simulink model "Lab1_works_ish"  (R2018a)
settings: Solver=VariableStepAuto  StartTime=0.0  StopTime=100  RelTol=1e-3
values from neighbouring files (symbols this model uses):
  Ac = [-(a*g*sqrt(2))/(2*sqrt((h10+h0)*g)*A) 0 ... (first row only)    [Lab1.m]    (also in LabB_FInal_version2.mat = [-0.0357235328446  0; 0.0357235328446  -0.0357235328446]; Untitled.m)
  Bc = [1/A ... (first row only)    [Lab1.m]    (also in LabB_FInal_version2.mat = [0.030303030303 0]; Untitled.m)
  C1 = [1 0]    [Lab1.m]    (also in LabB_FInal_version2.mat; Untitled.m)
  C2 = [0 1]    [Lab1.m]    (also in LabB_FInal_version2.mat; Untitled.m)
  K = K'    [Lab1.m]    (also in LabB_FInal_version2.mat = [5.99248777663 0.992989193414]; Untitled.m)
  v = 1:1:10    [Lab1.m]    (also in LabB_FInal_version2.mat = [1 2 3 4 5 6 7 8 9 10]; Untitled.m)
  vt = [21.18, 26.66 30.97, 34.28, 37.92, 39.73, 42.53, 45.45, 46.49, 47.67]    [Lab1.m]    (also in LabB_FInal_version2.mat = [21.18 26.66 30.97 34.28 37.92 39.73 42.53 45.45 46.49 47.67; Untitled.m)
settings Model: Creator=Scott  LastModifiedBy=oscbck-5

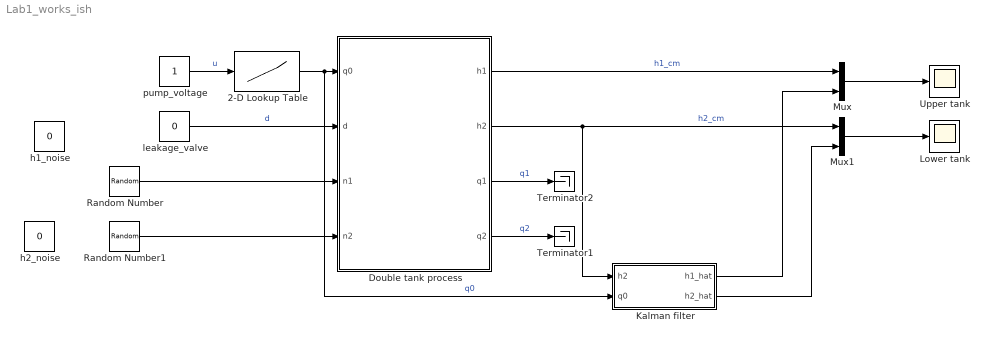
== system Lab1_works_ish ==
  2-D Lookup Table : Lookup_n-D  NumberOfTableDimensions=1  BreakpointsForDimension1=x  BreakpointsForDimension2=[1:3]  Table=y  RndMeth=Simplest  InputSameDT=on  mask{x=v, y=vt}
      mask prompts: x "Values on x-axis"; y "Values on y-axis"
  Double tank process : Subsystem  mask{At=33, Ao=0.17, hmax=15.5}
      mask prompts: At "Tank area (cm^2)"; Ao "Opening area (cm^2)"; hmax "Tank height (cm)"
      mask help: Double tank process parameters
  Kalman filter : Subsystem
  Lower tank : Scope
  Mux : Mux  Inputs=2
  Mux1 : Mux  Inputs=2
  Random Number : RandomNumber  Variance=0.1  SampleTime=0.1
  Random Number1 : RandomNumber  Variance=0.1  SampleTime=0.1
  Terminator1 : Terminator
  Terminator2 : Terminator
  Upper tank : Scope
  h1_noise : Constant  Value=0
  h2_noise : Constant  Value=0
  leakage_valve : Constant  Value=0
  pump_voltage : Constant
  wires:
  2-D Lookup Table/1 -> Kalman filter/2(q0), Double tank process/1(q0)  "q0"
  Double tank process/2(h2) -> Mux1/1, Kalman filter/1(h2)  "h2_cm"
  leakage_valve/1 -> Double tank process/2(d)  "d"
  pump_voltage/1 -> 2-D Lookup Table/1  "u"
  Double tank process/1(h1) -> Mux/1  "h1_cm"
  Double tank process/3(q1) -> Terminator2/1  "q1"
  Double tank process/4(q2) -> Terminator1/1  "q2"
  Mux/1 -> Upper tank/1
  Kalman filter/1(h1_hat) -> Mux/2
  Mux1/1 -> Lower tank/1
  Kalman filter/2(h2_hat) -> Mux1/2
  Random Number1/1 -> Double tank process/4(n2)
  Random Number/1 -> Double tank process/3(n1)

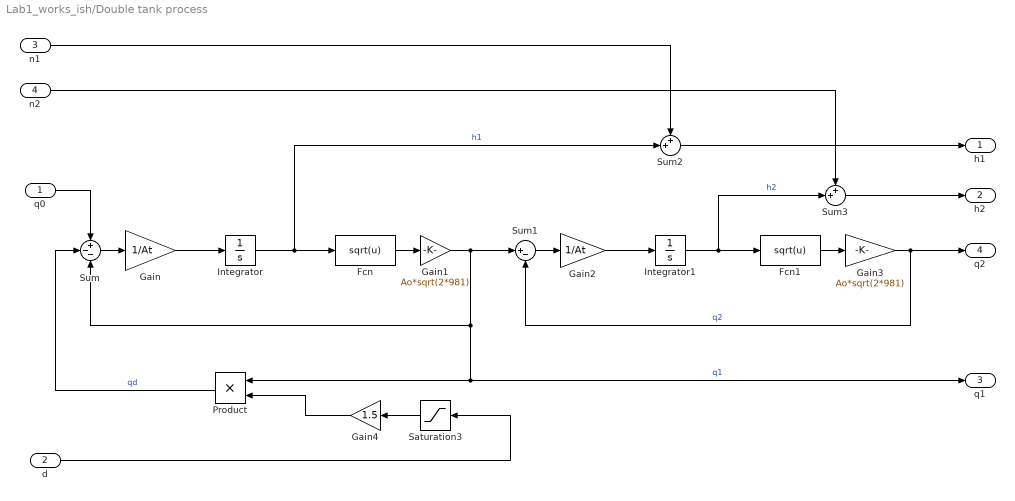
== system Lab1_works_ish/Double tank process ==
  q0 : Inport
  d : Inport  Port=2
  n1 : Inport  Port=3
  n2 : Inport  Port=4
  Fcn : Fcn  Expr=sqrt(u)
  Fcn1 : Fcn  Expr=sqrt(u)
  Gain : Gain  Gain=1/At
  Gain1 : Gain  Gain=Ao*sqrt(2*981)
  Gain2 : Gain  Gain=1/At
  Gain3 : Gain  Gain=Ao*sqrt(2*981)
  Gain4 : Gain  Gain=1.5
  Integrator : Integrator  LimitOutput=on  UpperSaturationLimit=hmax  LowerSaturationLimit=0
  Integrator1 : Integrator  LimitOutput=on  UpperSaturationLimit=hmax  LowerSaturationLimit=0
  Product : Product  RndMeth=Zero
  Saturation3 : Saturate  UpperLimit=1  LowerLimit=0
  Sum : Sum  Inputs=+--
  Sum1 : Sum  Inputs=|+-
  Sum2 : Sum  Inputs=++|
  Sum3 : Sum  Inputs=++|
  h1 : Outport
  h2 : Outport  Port=2
  q1 : Outport  Port=3
  q2 : Outport  Port=4
  wires:
  Sum/1 -> Gain/1
  Gain/1 -> Integrator/1
  Fcn/1 -> Gain1/1
  Gain1/1 -> Sum1/1, Product/1, q1/1, Sum/3  "q1"
  Sum1/1 -> Gain2/1
  Gain2/1 -> Integrator1/1
  Fcn1/1 -> Gain3/1
  Gain3/1 -> Sum1/2, q2/1  "q2"
  q0/1 -> Sum/1
  Integrator/1 -> Sum2/2, Fcn/1  "h1"
  Product/1 -> Sum/2  "qd"
  d/1 -> Saturation3/1
  Integrator1/1 -> Sum3/2, Fcn1/1  "h2"
  Saturation3/1 -> Gain4/1
  Gain4/1 -> Product/2
  Sum2/1 -> h1/1
  n1/1 -> Sum2/1
  Sum3/1 -> h2/1
  n2/1 -> Sum3/1

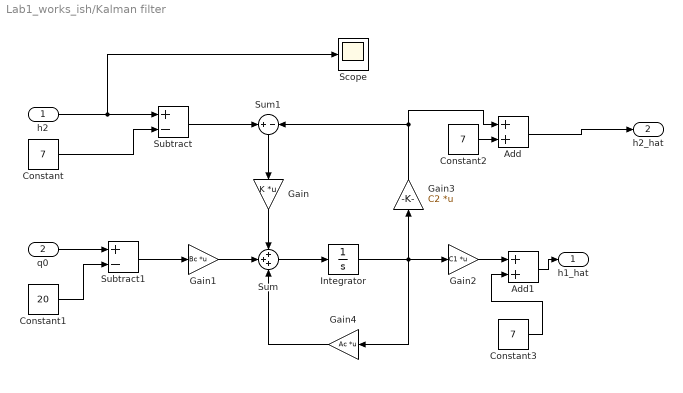
== system Lab1_works_ish/Kalman filter ==
  h2 : Inport
  q0 : Inport  Port=2
  Add : Sum
  Add1 : Sum
  Constant : Constant  Value=7
  Constant1 : Constant  Value=20
  Constant2 : Constant  Value=7
  Constant3 : Constant  Value=7
  Gain : Gain  Gain=K  Multiplication=Matrix(K*u)
  Gain1 : Gain  Gain=Bc  Multiplication=Matrix(K*u)
  Gain2 : Gain  Gain=C1  Multiplication=Matrix(K*u)
  Gain3 : Gain  Gain=C2  Multiplication=Matrix(K*u)
  Gain4 : Gain  Gain=Ac  Multiplication=Matrix(K*u)
  Integrator : Integrator
  Scope : Scope
  Subtract : Sum  Inputs=+-
  Subtract1 : Sum  Inputs=+-
  Sum : Sum  Inputs=+++
  Sum1 : Sum  Inputs=+|-
  h1_hat : Outport
  h2_hat : Outport  Port=2
  wires:
  Integrator/1 -> Gain4/1, Gain3/1, Gain2/1
  Sum/1 -> Integrator/1
  Gain2/1 -> Add1/1
  Sum1/1 -> Gain/1
  Gain/1 -> Sum/1
  Gain3/1 -> Add/1, Sum1/2
  Gain4/1 -> Sum/3
  Gain1/1 -> Sum/2
  h2/1 -> Scope/1, Subtract/1
  Subtract/1 -> Sum1/1
  Constant/1 -> Subtract/2
  q0/1 -> Subtract1/1
  Constant1/1 -> Subtract1/2
  Subtract1/1 -> Gain1/1
  Add/1 -> h2_hat/1
  Constant2/1 -> Add/2
  Constant3/1 -> Add1/2
  Add1/1 -> h1_hat/1
